simulink model "CRC_Test"  (R2019a)
settings: Solver=VariableStepAuto  StartTime=0.0  StopTime=1  RelTol=1e-3
values from neighbouring files (symbols this model uses):
  data_length = length(data)    [CRC_Generator.m]    (also in matlab.mat = 10)
  generate_polynomial = [1 0 1 1]    [matlab.mat]
libraries: commcrc2 x2, commutil2 x1, dspsrcs4 x1
settings Model: Creator=kaili  LastModifiedBy=kaili

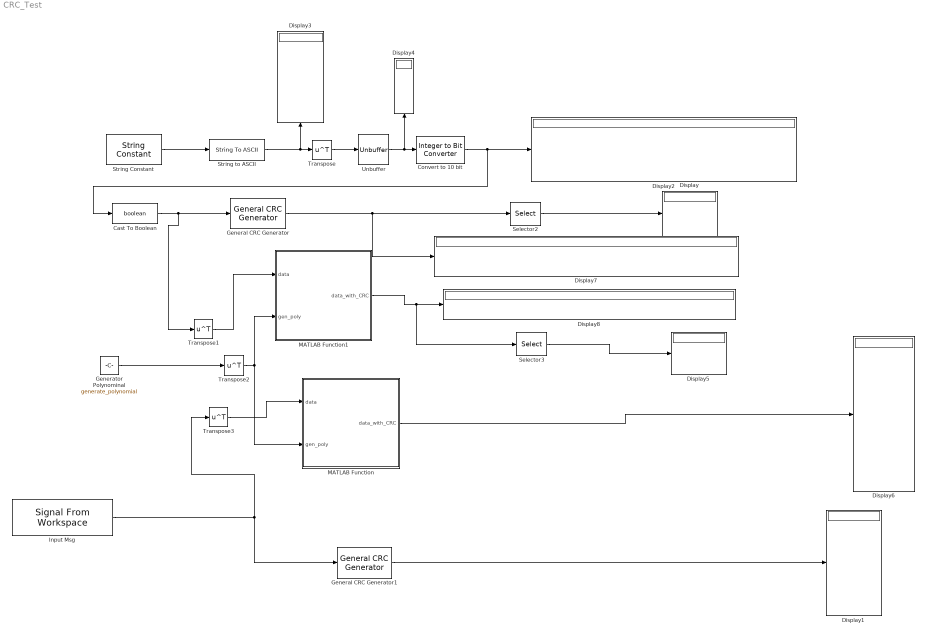
== system CRC_Test ==
  Cast To Boolean : DataTypeConversion  OutDataTypeStr=boolean
  Convert to 10 bit : commutil2/Integer to Bit Converter  nbits=10  signedInputValues=Unsigned  bitOrder=MSB first  outDtype=Inherit via internal rule
      settings: SourceProductName=Communications Toolbox
  Display{,1..8} (9 alike) : Display
  General CRC Generator : commcrc2/General CRC Generator  genPoly=generate_polynomial  iniStates=[ 0 ]  directMethod=off  reflectInputBytes=off  reflectChecksums=off  finalXOR=0  numChecksums=1
      settings: SourceProductName=Communications Toolbox  SourceProductBaseCode=CM
  General CRC Generator1 : commcrc2/General CRC Generator  genPoly=generate_polynomial  iniStates=[ 0 ]  directMethod=off  reflectInputBytes=off  reflectChecksums=off  finalXOR=0  numChecksums=1
      settings: SourceProductName=Communications Toolbox  SourceProductBaseCode=CM
  Generator Polynominal : Constant  Value=generate_polynomial
  "Input Msg " : dspsrcs4/Signal From Workspace  X=[1 1 1 1 0 1 ]  Ts=1  nsamps=6  OutputAfterFinalValue=Setting to zero  ignoreOrWarnInputAndFrameLengths=off  OutputFrames=off
  MATLAB Function : MATLAB Function  TreatAsAtomicUnit=on
  MATLAB Function1 : MATLAB Function  TreatAsAtomicUnit=on
  Selector2 : Selector  InputPortWidth=data_length+3  IndexOptions=Index vector (dialog)  Indices=[data_length+1:data_length+3]  OutputSizes=1
  Selector3 : Selector  InputPortWidth=10+3  IndexOptions=Index vector (dialog)  Indices=[data_length+1:data_length+3]  OutputSizes=1
  String Constant : StringConstant  String="\"K\""
  String to ASCII : StringToASCII
  Transpose{,1..3} (4 alike) : Math  Operator=transpose  SaturateOnIntegerOverflow=on
  Unbuffer : Unbuffer
  wires:
  "Input Msg "/1 -> General CRC Generator1/1, Transpose3/1
  General CRC Generator/1 -> Display7/1, Selector2/1
  Selector2/1 -> Display/1
  General CRC Generator1/1 -> Display1/1
  String to ASCII/1 -> Display3/1, Transpose/1
  String Constant/1 -> String to ASCII/1
  Unbuffer/1 -> Convert to 10 bit/1, Display4/1
  Convert to 10 bit/1 -> Cast To Boolean/1, Display2/1
  Transpose/1 -> Unbuffer/1
  Cast To Boolean/1 -> Transpose1/1, General CRC Generator/1
  Selector3/1 -> Display5/1
  Generator Polynominal/1 -> Transpose2/1
  MATLAB Function/1(data_with_CRC) -> Display6/1
  Transpose3/1 -> MATLAB Function/1(data)
  Transpose2/1 -> MATLAB Function/2(gen_poly), MATLAB Function1/2(gen_poly)
  Transpose1/1 -> MATLAB Function1/1(data)
  MATLAB Function1/1(data_with_CRC) -> Selector3/1, Display8/1

== matlab function CRC_Test/MATLAB Function1 ==
  data: data input; data_with_CRC output; gen_poly input
%data: row vector of logical 1 and 0 bits
% gen_poly: row vector  representing the polynom

function data_with_CRC = CRC_Generator(data,gen_poly)
data_length=length(data);
CRC_length = length(gen_poly)-1;
CRC_Code = logical(zeros(1,CRC_length));
index = 1;
zrs = logical(zeros(1,CRC_length+1));
data_append=[logical(data) zrs];
current_data = data_append(index:CRC_length+index);
tmp=zeros(CRC_length+1,1)';
tmp_index=1;
data_start=0;
to_add = 0;
while index <= data_length
    tmp = bitxor(logical(current_data),logical(gen_poly));
    tt=find(tmp~=0,1);
    tmp_index = tt(1);
    data_start = index+CRC_length+1;
    prev_index = index;
    index = index + tmp_index-1;
    to_add = tmp_index-1;
    if index > data_length
        tmp_curr = tmp(data_length-prev_index+2:end);
        current_data_ = [tmp_curr false(1,CRC_length+1-length(tmp_curr))];
        current_data = current_data_(1,1:CRC_length+1);
        break;
    else
        current_data_ = [tmp(tmp_index:end) data_append(data_start:data_start+to_add-1)];
        current_data = current_data_(1,1:CRC_length+1);
    end
end

CRC_Code = current_data(1:CRC_length);



data_with_CRC = logical([data, CRC_Code]);

== matlab function CRC_Test/MATLAB Function ==
  data: data input; data_with_CRC output; gen_poly input
%data: row vector of logical 1 and 0 bits
% gen_poly: row vector  representing the polynom

function data_with_CRC = CRC_Generator(data,gen_poly)
data_length=length(data);
CRC_length = length(gen_poly)-1;
CRC_Code = logical(zeros(1,CRC_length));
index = 1;
zrs = logical(zeros(1,CRC_length+1));
data_append=[logical(data) zrs];
current_data = data_append(index:CRC_length+index);
tmp=zeros(CRC_length+1,1)';
tmp_index=1;
data_start=0;
to_add = 0;
while index <= data_length
    tmp = bitxor(logical(current_data),logical(gen_poly));
    tt=find(tmp~=0,1);
    %TODO: solve the case when all tmp is 0 and tt == []
    tmp_index = tt(1);
    data_start = index+CRC_length+1;
    prev_index = index;
    index = index + tmp_index-1;
    to_add = tmp_index-1;
    if index > data_length
        tmp_curr = tmp(data_length-prev_index+2:end);
        current_data_ = [tmp_curr false(1,CRC_length+1-length(tmp_curr))];
        current_data = current_data_(1,1:CRC_length+1);
        break;
    else
        current_data_ = [tmp(tmp_index:end) data_append(data_start:data_start+to_add-1)];
        current_data = current_data_(1,1:CRC_length+1);
    end
end

CRC_Code = current_data(1:CRC_length);



data_with_CRC = logical([data, CRC_Code]);
